simulink subsystem "Modular_Motor"  (R2022b)
settings: Solver=VariableStepAuto  StartTime=0.0  StopTime=10.0  RelTol=1e-3
model mask{motor_model=0, initial_conditions=zeros(4,1), flux_weakening=on, coulomb_friction=on, stribeck_friction=on}
  mask prompts: motor_model "Motor Parameters struct:"; initial_conditions "Motor Initial Conditions:"; flux_weakening "Flux Weakening Effect:"; coulomb_friction "Coulomb Friction Effect:"; stribeck_friction "Stribeck Friction Effect:"
settings Model: Creator=gotta  LastModifiedBy=gotta

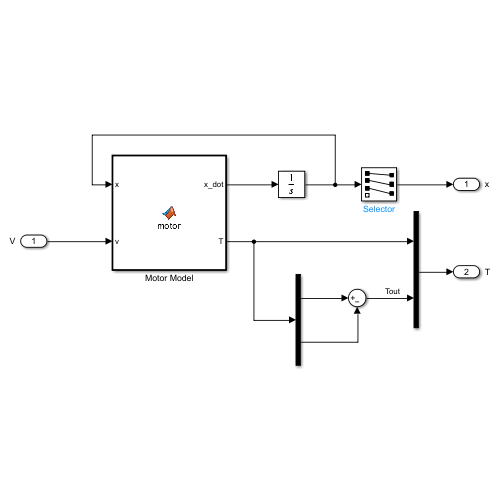
[thumbnail: Simulink's stored preview of the top-level diagram]
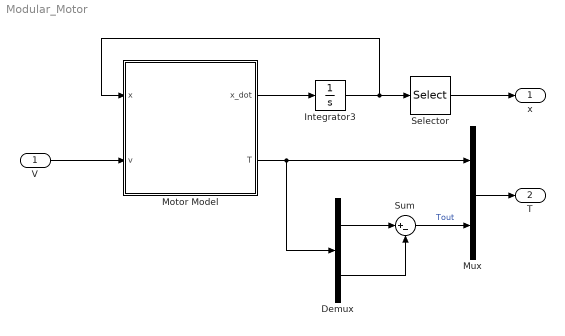
== system Modular_Motor ==
  V : Inport
  Demux : Demux  Outputs=2
  Integrator3 : Integrator  InitialCondition=initial_conditions
  Motor Model : MATLAB Function  TreatAsAtomicUnit=on
  Mux : Mux  Inputs=2
  Selector : Selector  InputPortWidth=4  IndexOptions=Index vector (dialog)  Indices=[1:3]  OutputSizes=1
  Sum : Sum  Inputs=|+-
  x : Outport
  T : Outport  Port=2
  wires:
  Integrator3/1 -> Motor Model/1(x), Selector/1
  Motor Model/1(x_dot) -> Integrator3/1
  V/1 -> Motor Model/2(v)
  Motor Model/2(T) -> Mux/1, Demux/1
  Selector/1 -> x/1
  Demux/1 -> Sum/1
  Demux/2 -> Sum/2
  Sum/1 -> Mux/2  "Tout"
  Mux/1 -> T/1

== matlab function Modular_Motor/Motor Model ==
  data: x input; v input; x_dot output; T output; motor_model parameter; flux_weakening parameter; coulomb_friction parameter; stribeck_friction parameter
function [x_dot, T] = motor(x, v, motor_model, flux_weakening, coulomb_friction, stribeck_friction)
%% Model Nonlinearities Selection

nl_options.flux = flux_weakening;
nl_options.coulomb = coulomb_friction;
nl_options.stribeck = stribeck_friction;


x_dot = motor_dynamics(x, v, motor_model, nl_options);

% Tm = (PHI_ws + Kphi)*x(3);
% Tf = s0*x(4) + s1*x_dot(4) + Be*x(2)/Kg;
% 
% T = [Tm, Tf];
T = [0, 0];
